simulink model "simTopLevel"  (R2016b)
settings: Solver=ode15s  StartTime=0.0  StopTime=2  RelTol=1e-3  EnableMultiTasking=on
InitFcn:
  | % minitaurParameters
model workspace (MAT data in the model file):
  IC = Simulink.Parameter
  IC.Value.Minitaur.IAq = -0.785398163397
  IC.Value.Minitaur.IAqDot = 0
  IC.Value.Minitaur.IBq = 0.785398163397
  IC.Value.Minitaur.IBqDot = 0
  IC.Value.Minitaur.IIAq = -0.785398163397
  IC.Value.Minitaur.IIAqDot = 0
  IC.Value.Minitaur.IIBq = 0.785398163397
  IC.Value.Minitaur.IIBqDot = 0
  IC.Value.Minitaur.IIIAq = -0.785398163397
  IC.Value.Minitaur.IIIAqDot = 0
  IC.Value.Minitaur.IIIBq = 0.785398163397
  IC.Value.Minitaur.IIIBqDot = 0
  IC.Value.Minitaur.IVAq = -0.785398163397
  IC.Value.Minitaur.IVAqDot = 0
  IC.Value.Minitaur.IVBq = 0.785398163397
  IC.Value.Minitaur.IVBqDot = 0
  IC.Value.Minitaur.ToeJointR = 1.57079632679
  IC.Value.Minitaur.ToeJointL = -1.57079632679
  IC.Value.Minitaur.Body.x = 0
  IC.Value.Minitaur.Body.y = -48
  IC.Value.Minitaur.Body.z = 0.7
  IC.Value.Minitaur.Body.xDot = 0
  IC.Value.Minitaur.Body.yDot = 0
  IC.Value.Minitaur.Body.zDot = 0
  IC.Value.Minitaur.Body.RotXZX = [0 3.14159265359 1.57079632679]
  IC.Value.Minitaur.Body.w = [0 0 0]
  IC.DataType = 'struct'
  IC.Dimensions = [1 1]
  controlParams = Simulink.Parameter
  controlParams.Value.jointPID.P = 6
  controlParams.Value.jointPID.I = 0.1
  controlParams.Value.jointPID.D = 0.07
  controlParams.Value.jointPID.N = 1000
  controlParams.Value.CPG.ForeRearLag = 1.57079632679
  controlParams.Value.CPG.Period = 1
  controlParams.Value.CPG.LRSyncFlag = 0
  controlParams.Value.FootImpedanceControl.r0 = -0.2
  controlParams.Value.FootImpedanceControl.rx = 0.04
  controlParams.Value.FootImpedanceControl.ry = 0.04
  controlParams.Value.FootImpedanceControl.thetaTilt = 0
  controlParams.DataType = 'struct'
  controlParams.Dimensions = [1 1]
  envParams = Simulink.Parameter
  envParams.Value.Ground.Width = 10
  envParams.Value.Ground.Length = 100
  envParams.Value.Ground.FrameDepth = 0.5
  envParams.Value.Contact.FootContactRadius = 0.0075
  envParams.Value.Contact.Stiffness = 10000
  envParams.Value.Contact.Damping = 1000
  envParams.Value.Contact.MuK = 0.75
  envParams.Value.Contact.MuS = 1
  envParams.Value.Contact.VelThresh = 0.01
  envParams.DataType = 'struct'
  envParams.Dimensions = [1 1]
  minitaurParams : Simulink.Parameter (value not decoded)
values from neighbouring files (symbols this model uses):
  controlParams = Simulink.Parameter(controlParams)    [minitaurParameters.m]
  envParams = Simulink.Parameter(envParams)    [minitaurParameters.m]
  IC = Simulink.Parameter(IC)    [minitaurParameters.m]
  minitaurParams = Simulink.Parameter(minitaurParams)    [minitaurParameters.m]
undefined symbols (not defined in the file or in its folder): Axis, Fn, ForeRearLag, Period, tau0, tau1, X, Y, Z
libraries: sm_lib x464, fl_lib x132, nesl_utility x41, Contact_Forces_Lib x28, simulink x13, simulink_extras x1
(part 1 of 13)
settings Model: SimulationMode=rapid-accelerator  Creator=Alexander  LastModifiedBy=Alexander
settings SolverCC: InitialStep=1e-12  MaxOrder=2  ZeroCrossAlgorithm=Adaptive  AlgebraicLoopSolver=LineSearch
settings DataIOCC: SaveFormat=StructureWithTime  SaveOutput=off  DSMLogging=off  SaveTime=off  SignalLoggingName=loggedSignals  ReturnWorkspaceOutputsName=simOut
settings OptimizationCC: DefaultParameterBehavior=Inlined  UseFloatMulNetSlope=on  InlineInvariantSignals=on  EfficientFloat2IntCast=on  EfficientMapNaN2IntZero=off  SimCompilerOptimization=on  AccelVerboseBuild=on
settings DebuggingCC: ReadBeforeWriteMsg=DisableAll  WriteAfterWriteMsg=DisableAll  WriteAfterReadMsg=DisableAll  MultiTaskDSMMsg=none  StrictBusMsg=ErrorOnBusTreatedAsVector  SFUnexpectedBacktrackingDiag=warning  SFNoUnconditionalDefaultTransitionDiag=warning  SFExecutionAtInitializationDiag=none
settings HardwareCC: TargetBitPerPointer=64  TargetBitPerSizeT=64  TargetBitPerPtrDiffT=64  TargetLongLongMode=on  TargetIntDivRoundTo=Zero  TargetEndianess=LittleEndian  TargetWordSize=64  TargetHWDeviceType=MATLAB Host
settings ModelReferenceCC: UpdateModelReferenceTargets=IfOutOfDate  ModelReferenceMinAlgLoopOccurrences=on
settings SFSimCC: SFSimEcho=off  SimBuildMode=sf_nonincremental_build
settings RTWCC: SystemTargetFile=rsim.tlc  TemplateMakefile=rsim_default_tmf  Description=Rapid Simulation Target  BuildConfiguration=Faster Runs  RTWCompilerOptimization=on
settings CodeAppCC: GenerateComments=off  MaxIdLength=128  SimulinkBlockComments=off
settings RSimTargetCC: TargetLangStandard=C99 (ISO)  ERTMultiwordTypeDef=System defined  ERTMultiwordLength=256  GeneratePreprocessorConditionals=Use local settings  CombineOutputUpdateFcns=on  MatFileLogging=off  SupportNonFinite=off  GRTInterface=off
settings ConfigComp: CovMetricSettings=dw  CovHtmlReporting=on  CovSaveCumulativeToWorkspaceVar=on  CovSaveSingleToWorkspaceVar=on  CovExternalEMLEnable=off
settings SimscapeCC: SimscapeLogSimulationStatistics=on  SimscapeLogLimitData=off
settings DiagnosticsConfigSet: SimMechanicsConflictingReferenceFrames=none  SimMechanicsRigidlyBoundBlock=none
settings ExplorerConfigSet: SimMechanicsOpenEditorOnUpdate=off  InternalSimMechanicsExplorerSettings="<ExplorerConfiguration><canonicalview>default</canonicalview><AnimationSetting><BasePlaybackSpeed>1.0</BasePlaybackSpeed><PlaybackSpeedFactor>0.125</PlaybackSpeedFactor></AnimationSetting><TilePanel><TileInfo><Tiles Columns=\"1\" Count=\"1\" Rows=\"1\"><Column Left=\"2\" Weight=\"1\"/><Column Left=\"1756\"/><Row Top=\"2\" Weight=\"1\"/><Row Top=\"912\"/><Tile Height=\"1\" Width=\"1\" X=\"0\" Y=\"0\"/></Tiles></TileInfo><SceneInfo><SceneViewer><BGColor><R>1</R><G>1</G><B>1</B></BGColor><Camera><DoPerspective>off</DoPerspective><Position><X>-52.933294827113023</X><Y>-19.442216136587813</Y><Z>35.583757754903054</Z></Position><Center><X>-14.397719012965357</X><Y>-39.827842104588491</Y><Z>10.080859987122921</Z></Center><Up><X>0.49923040919556116</X><Y>-0.12831156182763981</Y><Z>0.85691606452194846</Z></Up><ViewLimDist>1</ViewLimDist><YLim>0.49041337827292897</YLim><XLim>0.9498017148571154</XLim></Camera></SceneViewer></SceneInfo></TilePanel><MechEditorPanel><Cameras><Camera><Id>Camera1</Id><Value><Name>POV Camera</Name><NativeCamera><PositionTrackingFeature>POV_Camera.R</PositionTrackingFeature><CenterTrackingFeature>POV_Camera.R</CenterTrackingFeature><UpVectorTrackingFeature>POV_Camera.R</UpVectorTrackingFeature><CenterTrackingOrigin>off</CenterTrackingOrigin><CenterTrackingDirection>-Z</CenterTrackingDirection><UpVectorTrackingDirection>-Y</UpVectorTrackingDirection></NativeCamera></Value></Camera><Camera><Id>Camera2</Id><Value><Name>Side View</Name><NativeCamera><PositionTrackingFeature>Side_View_Camera.R</PositionTrackingFeature><CenterTrackingFeature>Body_Tracker.F</CenterTrackingFeature><UpVectorTrackingFeature>World1.W</UpVectorTrackingFeature><CenterTrackingOrigin>on</CenterTrackingOrigin><UpVectorTrackingDirection>+Z</UpVectorTrackingDirection></NativeCamera></Value></Camera></Cameras><GfxPanelCameraMap/><VideoCreator><PlaybackSpeedRatio>1.0</PlaybackSpeedRatio><FrameRate>30</FrameRate><VideoFormat>Motion JPEG AVI</VideoFormat><FrameSize>auto</FrameSize></VideoCreator></MechEditorPanel></ExplorerConfiguration>"

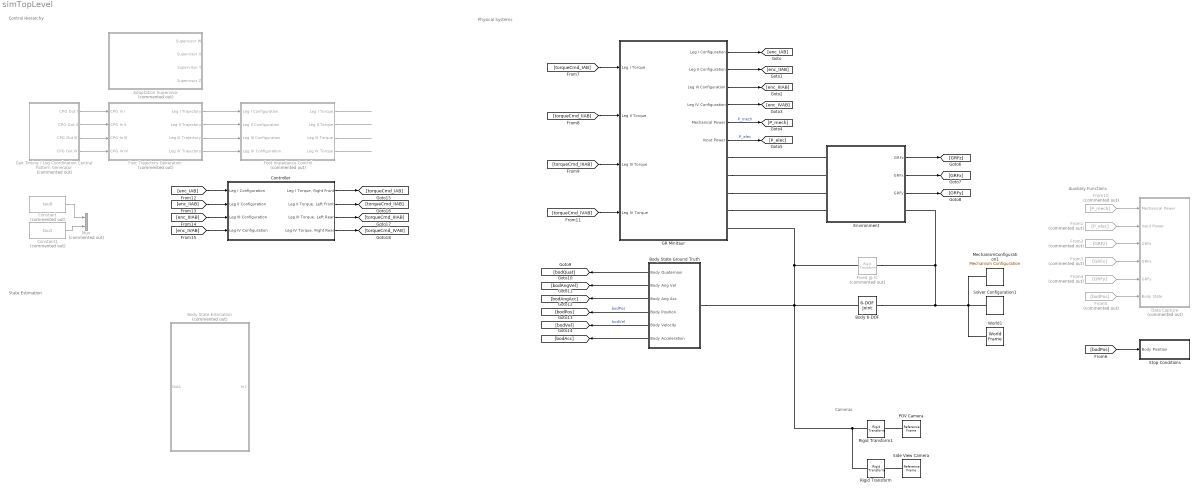
== system simTopLevel ==
  note: Physical Systems
  note: Control Hierarchy
  note: Auxiliary Functions
  note: Cameras
  note: State Estimation
  Adaptation Supervisor : Subsystem  Commented=on
  Body 6-DOF : sm_lib/Joints/6-DOF Joint  SenseConstraintForce=off  SenseConstraintForceX=off  SenseConstraintForceY=off  SenseConstraintForceZ=off  SenseConstraintTorque=off  SenseConstraintTorqueX=off  SenseConstraintTorqueY=off  SenseConstraintTorqueZ=off  SenseTotalForce=off  SenseTotalForceX=off  SenseTotalForceY=off  SenseTotalForceZ=off  SenseTotalTorque=off  SenseTotalTorqueX=off  SenseTotalTorqueY=off  SenseTotalTorqueZ=off  CompositeWrenchDir=FollowerOnBase  CompositeWrenchFrame=BaseFrame  PxEquilibriumPosition=0  PxEquilibriumPositionUnits=m  PxSpringStiffness=0  PxSpringStiffnessUnits=N/m  PxDampingCoefficient=0  PxDampingCoefficientUnits=N/(m/s)  PxTorqueActuationMode=NoTorque  PxMotionActuationMode=ComputedMotion  PxSensePosition=off  PxSenseVelocity=off  PxSenseAcceleration=off  PxSenseTorqueForce=off  PxPositionTargetSpecify=on  PxPositionTargetPriority=High  PxPositionTargetValue=IC.Minitaur.Body.x  PxPositionTargetValueUnits=m  PxVelocityTargetSpecify=on  PxVelocityTargetPriority=High  PxVelocityTargetValue=IC.Minitaur.Body.xDot  PxVelocityTargetValueUnits=m/s  PyEquilibriumPosition=0  PyEquilibriumPositionUnits=m  PySpringStiffness=0  PySpringStiffnessUnits=N/m  PyDampingCoefficient=0  PyDampingCoefficientUnits=N/(m/s)  PyTorqueActuationMode=NoTorque  PyMotionActuationMode=ComputedMotion  PySensePosition=off  PySenseVelocity=off  PySenseAcceleration=off  PySenseTorqueForce=off  PyPositionTargetSpecify=on  PyPositionTargetPriority=High  PyPositionTargetValue=IC.Minitaur.Body.y  PyPositionTargetValueUnits=m  PyVelocityTargetSpecify=on  PyVelocityTargetPriority=High  PyVelocityTargetValue=IC.Minitaur.Body.yDot  PyVelocityTargetValueUnits=m/s  PzEquilibriumPosition=1  PzEquilibriumPositionUnits=m  PzSpringStiffness=0  PzSpringStiffnessUnits=N/m  PzDampingCoefficient=0  PzDampingCoefficientUnits=N/(m/s)  PzTorqueActuationMode=NoTorque  PzMotionActuationMode=ComputedMotion  PzSensePosition=off  PzSenseVelocity=off  PzSenseAcceleration=off  PzSenseTorqueForce=off  PzPositionTargetSpecify=on  PzPositionTargetPriority=High  PzPositionTargetValue=IC.Minitaur.Body.z  PzPositionTargetValueUnits=m  PzVelocityTargetSpecify=on  PzVelocityTargetPriority=High  PzVelocityTargetValue=IC.Minitaur.Body.zDot  PzVelocityTargetValueUnits=m/s  SphDefPosRotationMethod=None  SphDefPosRotationAngleUnits=deg  SphDefPosRotationStandardAxis=+Z  SphDefPosRotationAngle=0.0  SphDefPosRotationArbitraryAxis=[0 0 1]  SphDefPosFollAlignAxisA=+X  SphDefPosBaseAlignAxisA=+Y  SphDefPosFollAlignAxisB=+Y  SphDefPosBaseAlignAxisB=+Z  SphDefPosRotationSequenceAxes=FollowerAxes  SphDefPosRotationSequence=XYX  SphDefPosRotationSequenceAngles=[0 0 0]  SphDefPosRotationSequenceAnglesUnits=deg  SphDefPosRotationMatrix=[1 0 0; 0 1 0; 0 0 1]  SphEqPosRotationMethod=None  SphEqPosRotationAngleUnits=deg  SphEqPosRotationStandardAxis=+Z  SphEqPosRotationAngle=0.0  SphEqPosRotationArbitraryAxis=[0 0 1]  SphEqPosFollAlignAxisA=+X  SphEqPosBaseAlignAxisA=+Y  SphEqPosFollAlignAxisB=+Y  SphEqPosBaseAlignAxisB=+Z  SphEqPosRotationSequenceAxes=FollowerAxes  SphEqPosRotationSequence=XYX  SphEqPosRotationSequenceAngles=[0 0 0]  SphEqPosRotationSequenceAnglesUnits=deg  SphEqPosRotationMatrix=[1 0 0; 0 1 0; 0 0 1]  SphSpringStiffness=0  SphSpringStiffnessUnits=N*m/deg  SphDampingCoefficient=0  SphDampingCoefficientUnits=N*m/(deg/s)  SphActuateTorqueX=off  SphActuateTorqueY=off  SphActuateTorqueZ=off  SphActuateTorque=off  SphTorqueActuationMode=NoTorque  SphMotionActuationMode=ComputedMotion  SphActuationFrame=BaseFrame  SphSensePosition=off  SphSenseVelocityX=off  SphSenseVelocityY=off  SphSenseVelocityZ=off  SphSenseVelocity=off  SphSenseAccelerationX=off  SphSenseAccelerationY=off  SphSenseAccelerationZ=off  SphSenseAcceleration=off  SphSenseTorqueX=off  SphSenseTorqueY=off  SphSenseTorqueZ=off  SphSenseTorqueForce=off  SphSensingFrame=BaseFrame  SphPositionTargetRotationMethod=RotationSequence  SphPositionTargetRotationAngleUnits=deg  SphPositionTargetRotationStandardAxis=+Z  SphPositionTargetRotationAngle=0.0  SphPositionTargetRotationArbitraryAxis=[0 0 1]  SphPositionTargetFollAlignAxisA=+X  SphPositionTargetBaseAlignAxisA=+Y  SphPositionTargetFollAlignAxisB=+Y  SphPositionTargetBaseAlignAxisB=+Z  SphPositionTargetRotationSequenceAxes=BaseAxes  SphPositionTargetRotationSequence=XZX  SphPositionTargetRotationSequenceAngles=IC.Minitaur.Body.RotXZX  SphPositionTargetRotationSequenceAnglesUnits=rad  SphPositionTargetRotationMatrix=[1 0 0; 0 1 0; 0 0 1]  SphPositionTargetSpecify=on  SphPositionTargetPriority=High  SphVelocityTargetValue=IC.Minitaur.Body.w  SphVelocityTargetValueUnits=rad/s  SphVelocityTargetSpecify=on  SphVelocityTargetPriority=High  SphVelocityTargetInFollowerFrame=off
  Body State Estimation : Subsystem  Commented=on
  Body State Ground Truth : Subsystem
  Constant : Constant  Commented=on  Value=tau0
  Constant1 : Constant  Commented=on  Value=tau1
  Controller : Subsystem
  Data Capture : Subsystem  Commented=on
  Environment : Subsystem
  Fixed @ IC : sm_lib/Frames and Transforms/Rigid Transform  Commented=on  TranslationMethod=Cartesian  TranslationStandardOffset=0  TranslationLengthUnit=m  TranslationStandardAxis=+Z  TranslationCartesianOffset=[IC.Minitaur.Body.x IC.Minitaur.Body.y IC.Minitaur.Body.z + 0.5]  TranslationROffset=0  TranslationROffsetUnits=m  TranslationZOffset=0  TranslationZOffsetUnits=m  TranslationThetaOffset=0  TranslationThetaOffsetUnits=deg  RotationMethod=RotationSequence  RotationAngleUnits=deg  RotationStandardAxis=+Z  RotationAngle=0.0  RotationArbitraryAxis=[0 0 1]  FollAlignAxisA=+X  BaseAlignAxisA=+Y  FollAlignAxisB=+Y  BaseAlignAxisB=+Z  RotationSequenceAxes=BaseAxes  RotationSequence=XZX  RotationSequenceAngles=IC.Minitaur.Body.RotXZX  RotationSequenceAnglesUnits=rad  RotationMatrix=[1 0 0; 0 1 0; 0 0 1]
  Foot Impedance Control : Subsystem  Commented=on
  Foot Trajectory Generation : Subsystem  Commented=on
  From1 : From  Commented=on  GotoTag=P_elec
  From10 : From  Commented=on  GotoTag=P_mech
  From2 : From  Commented=on  GotoTag=GRFz
  From3 : From  Commented=on  GotoTag=GRFx
  From4 : From  Commented=on  GotoTag=GRFy
  From5 : From  Commented=on  GotoTag=bodPos
  GR Minitaur : Subsystem
  Gait Timing / Leg Coordination Central Pattern Generator : Subsystem  Commented=on
  MechanismConfiguration1 : sm_lib/Utilities/Mechanism Configuration  UniformGravity=Constant  GravityVector="[0  0 -9.81]"  GravityUnits=m/s^2  LinearizationDelta=0.001
  Mux : Mux  Commented=on  Inputs=2
  POV Camera : sm_lib/Frames and Transforms/Reference Frame
  Rigid Transform : sm_lib/Frames and Transforms/Rigid Transform  TranslationMethod=Cartesian  TranslationStandardOffset=envParams.Ground.FrameDepth/2  TranslationLengthUnit=m  TranslationStandardAxis=+X  TranslationCartesianOffset=[-1 0 0]  TranslationROffset=0  TranslationROffsetUnits=m  TranslationZOffset=0  TranslationZOffsetUnits=m  TranslationThetaOffset=0  TranslationThetaOffsetUnits=deg  RotationMethod=None  RotationAngleUnits=deg  RotationStandardAxis=+Z  RotationAngle=0.0  RotationArbitraryAxis=[0 0 1]  FollAlignAxisA=+X  BaseAlignAxisA=+Y  FollAlignAxisB=+Y  BaseAlignAxisB=+Z  RotationSequenceAxes=FollowerAxes  RotationSequence=XYX  RotationSequenceAngles=[0 0 0]  RotationSequenceAnglesUnits=deg  RotationMatrix=[1 0 0; 0 1 0; 0 0 1]
  Rigid Transform1 : sm_lib/Frames and Transforms/Rigid Transform  TranslationMethod=Cartesian  TranslationStandardOffset=0  TranslationLengthUnit=m  TranslationStandardAxis=+Z  TranslationCartesianOffset=[0 -0.1 -0.125]  TranslationROffset=0  TranslationROffsetUnits=m  TranslationZOffset=0  TranslationZOffsetUnits=m  TranslationThetaOffset=0  TranslationThetaOffsetUnits=deg  RotationMethod=None  RotationAngleUnits=deg  RotationStandardAxis=+Z  RotationAngle=0.0  RotationArbitraryAxis=[0 0 1]  FollAlignAxisA=+X  BaseAlignAxisA=+Y  FollAlignAxisB=+Y  BaseAlignAxisB=+Z  RotationSequenceAxes=FollowerAxes  RotationSequence=XYX  RotationSequenceAngles=[0 0 0]  RotationSequenceAnglesUnits=deg  RotationMatrix=[1 0 0; 0 1 0; 0 0 1]
  Side View Camera : sm_lib/Frames and Transforms/Reference Frame
  Solver Configuration1 : nesl_utility/Solver Configuration  PhysicalDomain=network_engine_domain  SubClassName=solver  LeftPortType=input  RightPortType=generic  Accelerate=off  Tones=[]  Harmonics=[]  SimulateNoise=off  Profile=off  UseLocalSampling=off  EnableSwitchedLinearOptims=on  FrequencyDomain=off  UseCCode=off  RelTol=0.001  AbsTol=1e-06  MinStep=1e-09  ToWorkspace=off  RevertToSquareIcSolve=off  NumHomotopyIterations=100  PhasorMode=off  PhasorModeNumHarmonics=1  OverrideAbsTol=off  DoDC=off  ResidualTolerance=1e-09  UseLocalSolver=off  LocalSolverChoice=NE_BACKWARD_EULER_ADVANCER  LocalSolverSampleTime=0.001  DoFixedCost=off  MaxNonlinIter=3  MaxModeIter=2  LinearAlgebra=Sparse  DelaysMemoryBudget=1024  AutomaticFiltering=on  FilteringTimeConstant=0.001
  Stop Conditions : Subsystem
  World1 : sm_lib/Frames and Transforms/World Frame
  wires:
  GR Minitaur/1(Leg I Configuration) -> [enc_IAB]
  GR Minitaur/2(Leg II Configuration) -> [enc_IIAB]
  GR Minitaur/3(Leg III Configuration) -> [enc_IIIAB]
  GR Minitaur/4(Leg IV Configuration) -> [enc_IVAB]
  GR Minitaur/5(Mechanical Power) -> [P_mech]  "P_mech"
  GR Minitaur/6(Input Power) -> [P_elec]  "P_elec"
  From10/1 -> Data Capture/1(Mechanical Power)
  From1/1 -> Data Capture/2(Input Power)
  From2/1 -> Data Capture/3(GRFz)
  From3/1 -> Data Capture/4(GRFx)
  From4/1 -> Data Capture/5(GRFy)
  From5/1 -> Data Capture/6(Body State)
  Environment/1(GRFz) -> [GRFz]
  Environment/2(GRFx) -> [GRFx]
  Environment/3(GRFy) -> [GRFy]
  [bodPos] -> Stop Conditions/1(Body Position)
  [torqueCmd_IAB] -> GR Minitaur/1(Leg I Torque)
  [torqueCmd_IIAB] -> GR Minitaur/2(Leg II Torque)
  [torqueCmd_IIIAB] -> GR Minitaur/3(Leg III Torque)
  [torqueCmd_IVAB] -> GR Minitaur/4(Leg IV Torque)
  Body State Ground Truth/1(Body Quaternion) -> [bodQuat]
  Body State Ground Truth/2(Body Ang Vel) -> [bodAngVel]
  Body State Ground Truth/3(Body Ang Acc) -> [bodAngAcc]
  Body State Ground Truth/5(Body Velocity) -> [bodVel]  "bodVel"
  Body State Ground Truth/6(Body Acceleration) -> [bodAcc]
  Body State Ground Truth/4(Body Position) -> [bodPos]  "bodPos"
  Gait Timing / Leg Coordination Central Pattern Generator/1(CPG Out I) -> Foot Trajectory Generation/1(CPG In I)
  Gait Timing / Leg Coordination Central Pattern Generator/2(CPG Out II) -> Foot Trajectory Generation/2(CPG In II)
  Gait Timing / Leg Coordination Central Pattern Generator/3(CPG Out III) -> Foot Trajectory Generation/3(CPG In III)
  Gait Timing / Leg Coordination Central Pattern Generator/4(CPG Out IV) -> Foot Trajectory Generation/4(CPG In IV)
  Foot Trajectory Generation/1(Leg I Trajectory) -> Foot Impedance Control/1(Leg I Configuration)
  Foot Trajectory Generation/2(Leg II Trajectory) -> Foot Impedance Control/2(Leg II Configuration)
  Foot Trajectory Generation/3(Leg III Trajectory) -> Foot Impedance Control/3(Leg III Configuration)
  Foot Trajectory Generation/4(Leg IV Trajectory) -> Foot Impedance Control/4(Leg IV Configuration)
  Foot Impedance Control/1(Leg I Torque) -> ?
  Foot Impedance Control/2(Leg II Torque) -> ?
  Foot Impedance Control/4(Leg IV Torque) -> ?
  Foot Impedance Control/3(Leg III Torque) -> ?
  Constant1/1 -> Mux/2
  Constant/1 -> Mux/1
  Controller/1("Leg I Torque, Right Front") -> [torqueCmd_IAB]
  Controller/2("Leg II Torque, Left Front") -> [torqueCmd_IIAB]
  Controller/4("Leg IV Torque, Right Rear") -> [torqueCmd_IVAB]
  Controller/3("Leg III Torque, Left Rear") -> [torqueCmd_IIIAB]
  [enc_IAB] -> Controller/1(Leg I Configuration)
  [enc_IIAB] -> Controller/2(Leg II Configuration)
  [enc_IIIAB] -> Controller/3(Leg III Configuration)
  [enc_IVAB] -> Controller/4(Leg IV Configuration)
  connections:
  MechanismConfiguration1/RConn1 -- Solver Configuration1/RConn1 -- World1/RConn1 -- Fixed @ IC/LConn1 -- Environment/RConn1 -- Body 6-DOF/LConn1
  GR Minitaur/RConn4 -- Environment/LConn4
  GR Minitaur/RConn3 -- Environment/LConn3
  GR Minitaur/RConn2 -- Environment/LConn2
  GR Minitaur/RConn1 -- Environment/LConn1
  Rigid Transform/LConn1 -- Body State Ground Truth/LConn1 -- GR Minitaur/RConn5 -- Fixed @ IC/RConn1 -- Body 6-DOF/RConn1 -- Rigid Transform1/LConn1
  Side View Camera/RConn1 -- Rigid Transform/RConn1
  POV Camera/RConn1 -- Rigid Transform1/RConn1

== system simTopLevel/Adaptation Supervisor ==
  Constant{,1..3} (4 alike) : Constant
  Supervisor W : Outport
  Supervisor X : Outport  Port=2
  Supervisor Y : Outport  Port=3
  Supervisor Z : Outport  Port=4
  wires:
  Constant/1 -> Supervisor W/1
  Constant3/1 -> Supervisor Z/1
  Constant2/1 -> Supervisor Y/1
  Constant1/1 -> Supervisor X/1

== system simTopLevel/Body State Estimation ==
  In1 : Inport
  Out1 : Outport
  wires:
  In1/1 -> Out1/1

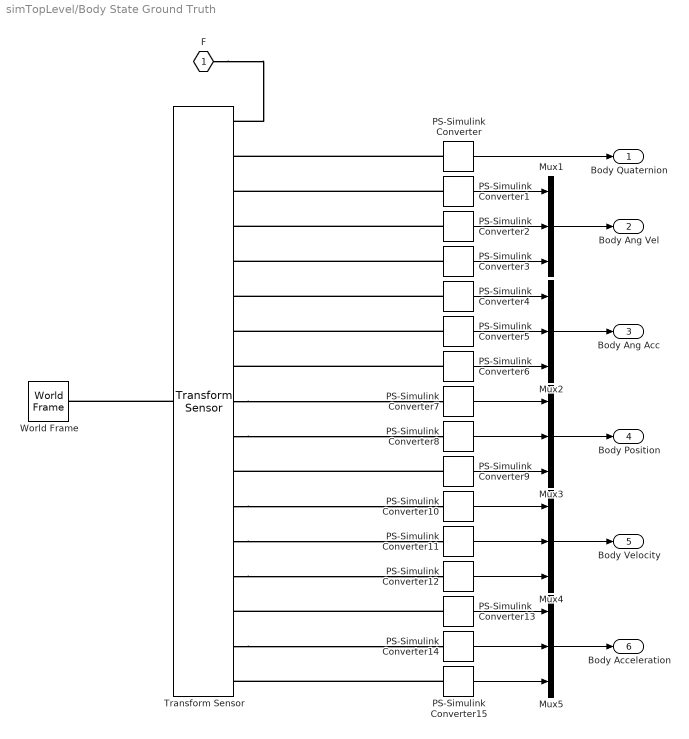
== system simTopLevel/Body State Ground Truth ==
  Mux{1..5} (5 alike) : Mux  Inputs=3
  PS-Simulink Converter : nesl_utility/PS-Simulink Converter  PhysicalDomain=network_engine_domain  SubClassName=ps_output  LeftPortType=input  RightPortType=output  PseudoPeriodic=off  Frequencies=[]  Unit=1  AffineConversion=off
  PS-Simulink Converter1 : nesl_utility/PS-Simulink Converter  PhysicalDomain=network_engine_domain  SubClassName=ps_output  LeftPortType=input  RightPortType=output  PseudoPeriodic=off  Frequencies=[]  Unit=rad/s  AffineConversion=off
  PS-Simulink Converter10 : nesl_utility/PS-Simulink Converter  PhysicalDomain=network_engine_domain  SubClassName=ps_output  LeftPortType=input  RightPortType=output  PseudoPeriodic=off  Frequencies=[]  Unit=m/s  AffineConversion=off
  PS-Simulink Converter11 : nesl_utility/PS-Simulink Converter  PhysicalDomain=network_engine_domain  SubClassName=ps_output  LeftPortType=input  RightPortType=output  PseudoPeriodic=off  Frequencies=[]  Unit=m/s  AffineConversion=off
  PS-Simulink Converter12 : nesl_utility/PS-Simulink Converter  PhysicalDomain=network_engine_domain  SubClassName=ps_output  LeftPortType=input  RightPortType=output  PseudoPeriodic=off  Frequencies=[]  Unit=m/s  AffineConversion=off
  PS-Simulink Converter13 : nesl_utility/PS-Simulink Converter  PhysicalDomain=network_engine_domain  SubClassName=ps_output  LeftPortType=input  RightPortType=output  PseudoPeriodic=off  Frequencies=[]  Unit=m/s^2  AffineConversion=off
  PS-Simulink Converter14 : nesl_utility/PS-Simulink Converter  PhysicalDomain=network_engine_domain  SubClassName=ps_output  LeftPortType=input  RightPortType=output  PseudoPeriodic=off  Frequencies=[]  Unit=m/s^2  AffineConversion=off
  PS-Simulink Converter15 : nesl_utility/PS-Simulink Converter  PhysicalDomain=network_engine_domain  SubClassName=ps_output  LeftPortType=input  RightPortType=output  PseudoPeriodic=off  Frequencies=[]  Unit=m/s^2  AffineConversion=off
  PS-Simulink Converter2 : nesl_utility/PS-Simulink Converter  PhysicalDomain=network_engine_domain  SubClassName=ps_output  LeftPortType=input  RightPortType=output  PseudoPeriodic=off  Frequencies=[]  Unit=rad/s  AffineConversion=off
  PS-Simulink Converter3 : nesl_utility/PS-Simulink Converter  PhysicalDomain=network_engine_domain  SubClassName=ps_output  LeftPortType=input  RightPortType=output  PseudoPeriodic=off  Frequencies=[]  Unit=rad/s  AffineConversion=off
  PS-Simulink Converter4 : nesl_utility/PS-Simulink Converter  PhysicalDomain=network_engine_domain  SubClassName=ps_output  LeftPortType=input  RightPortType=output  PseudoPeriodic=off  Frequencies=[]  Unit=rad/s^2  AffineConversion=off
  PS-Simulink Converter5 : nesl_utility/PS-Simulink Converter  PhysicalDomain=network_engine_domain  SubClassName=ps_output  LeftPortType=input  RightPortType=output  PseudoPeriodic=off  Frequencies=[]  Unit=rad/s^2  AffineConversion=off
  PS-Simulink Converter6 : nesl_utility/PS-Simulink Converter  PhysicalDomain=network_engine_domain  SubClassName=ps_output  LeftPortType=input  RightPortType=output  PseudoPeriodic=off  Frequencies=[]  Unit=rad/s^2  AffineConversion=off
  PS-Simulink Converter7 : nesl_utility/PS-Simulink Converter  PhysicalDomain=network_engine_domain  SubClassName=ps_output  LeftPortType=input  RightPortType=output  PseudoPeriodic=off  Frequencies=[]  Unit=m  AffineConversion=off
  PS-Simulink Converter8 : nesl_utility/PS-Simulink Converter  PhysicalDomain=network_engine_domain  SubClassName=ps_output  LeftPortType=input  RightPortType=output  PseudoPeriodic=off  Frequencies=[]  Unit=m  AffineConversion=off
  PS-Simulink Converter9 : nesl_utility/PS-Simulink Converter  PhysicalDomain=network_engine_domain  SubClassName=ps_output  LeftPortType=input  RightPortType=output  PseudoPeriodic=off  Frequencies=[]  Unit=m  AffineConversion=off
  Transform Sensor : sm_lib/Frames and Transforms/Transform Sensor  MeasurementFrame=World  SenseAngle=off  SenseAxis=off  SenseAngle1=off  SenseAngle2=off  SenseAngle3=off  SenseQ=on  SenseR=off  SenseOmegaX=on  SenseOmegaY=on  SenseOmegaZ=on  SenseOmega1=off  SenseOmega2=off  SenseOmega3=off  SenseQDot=off  SenseRDot=off  SenseAlphaX=on  SenseAlphaY=on  SenseAlphaZ=on  SenseAlpha1=off  SenseAlpha2=off  SenseAlpha3=off  SenseQDDot=off  SenseRDDot=off  SenseX=on  SenseY=on  SenseZ=on  SenseRad=off  SenseAzim=off  SenseDist=off  SenseInc=off  SenseXDot=on  SenseYDot=on  SenseZDot=on  SenseRadDot=off  SenseAzimDot=off  SenseDistDot=off  SenseIncDot=off  SenseXDDot=on  SenseYDDot=on  SenseZDDot=on  SenseRadDDot=off  SenseAzimDDot=off  SenseDistDDot=off  SenseIncDDot=off
  World Frame : sm_lib/Frames and Transforms/World Frame
  F : PMIOPort  Port=1  Side=Left
  Body Quaternion : Outport
  Body Ang Vel : Outport  Port=2
  Body Ang Acc : Outport  Port=3
  Body Position : Outport  Port=4
  Body Velocity : Outport  Port=5
  Body Acceleration : Outport  Port=6
  wires:
  PS-Simulink Converter3/1 -> Mux1/3
  PS-Simulink Converter2/1 -> Mux1/2
  PS-Simulink Converter1/1 -> Mux1/1
  PS-Simulink Converter/1 -> Body Quaternion/1
  Mux1/1 -> Body Ang Vel/1
  PS-Simulink Converter4/1 -> Mux2/1
  PS-Simulink Converter5/1 -> Mux2/2
  Mux2/1 -> Body Ang Acc/1
  PS-Simulink Converter6/1 -> Mux2/3
  PS-Simulink Converter7/1 -> Mux3/1
  PS-Simulink Converter8/1 -> Mux3/2
  PS-Simulink Converter9/1 -> Mux3/3
  Mux3/1 -> Body Position/1
  PS-Simulink Converter10/1 -> Mux4/1
  PS-Simulink Converter11/1 -> Mux4/2
  PS-Simulink Converter12/1 -> Mux4/3
  Mux4/1 -> Body Velocity/1
  PS-Simulink Converter13/1 -> Mux5/1
  PS-Simulink Converter14/1 -> Mux5/2
  PS-Simulink Converter15/1 -> Mux5/3
  Mux5/1 -> Body Acceleration/1
  connections:
  PS-Simulink Converter1/LConn1 -- Transform Sensor/RConn3
  PS-Simulink Converter5/LConn1 -- Transform Sensor/RConn7
  PS-Simulink Converter4/LConn1 -- Transform Sensor/RConn6
  F/RConn1 -- Transform Sensor/RConn1
  PS-Simulink Converter/LConn1 -- Transform Sensor/RConn2
  Transform Sensor/LConn1 -- World Frame/RConn1
  PS-Simulink Converter2/LConn1 -- Transform Sensor/RConn4
  PS-Simulink Converter3/LConn1 -- Transform Sensor/RConn5
  PS-Simulink Converter6/LConn1 -- Transform Sensor/RConn8
  Transform Sensor/RConn9 -- PS-Simulink Converter7/LConn1
  PS-Simulink Converter9/LConn1 -- Transform Sensor/RConn11
  Transform Sensor/RConn10 -- PS-Simulink Converter8/LConn1
  Transform Sensor/RConn12 -- PS-Simulink Converter10/LConn1
  Transform Sensor/RConn13 -- PS-Simulink Converter11/LConn1
  Transform Sensor/RConn14 -- PS-Simulink Converter12/LConn1
  PS-Simulink Converter13/LConn1 -- Transform Sensor/RConn15
  PS-Simulink Converter15/LConn1 -- Transform Sensor/RConn17
  Transform Sensor/RConn16 -- PS-Simulink Converter14/LConn1

== system simTopLevel/Controller ==
  Leg I Configuration : Inport  PortDimensions=2
  Leg II Configuration : Inport  Port=2  PortDimensions=2
  Leg III Configuration : Inport  Port=3  PortDimensions=2
  Leg IV Configuration : Inport  Port=4  PortDimensions=2
  Subsystem1 : Subsystem
  Subsystem2 : Subsystem
  Subsystem3 : Subsystem
  Subsystem4 : Subsystem
  Trajectory Planner : Subsystem
  "Leg I Torque, Right Front" : Outport
  "Leg II Torque, Left Front" : Outport  Port=2
  "Leg III Torque, Left Rear" : Outport  Port=3
  "Leg IV Torque, Right Rear" : Outport  Port=4
  wires:
  Trajectory Planner/1(Foot I Trajectory [psi L]) -> Subsystem4/1(Path Trajectory)
  Leg I Configuration/1 -> Subsystem4/2(Current leg state)  "[theta_AI theta_BI] Nm"
  Subsystem4/1(Leg Torque) -> "Leg I Torque, Right Front"/1
  Trajectory Planner/2(Foot II Trajectory [psi L]) -> Subsystem1/1(Path Trajectory)
  Trajectory Planner/3(Foot III Trajectory [psi L]) -> Subsystem2/1(Path Trajectory)
  Trajectory Planner/4(Foot IV Trajectory [psi L]) -> Subsystem3/1(Path Trajectory)
  Leg II Configuration/1 -> Subsystem1/2(Current leg state)  "[Tau_IIA Tau_IIB] Nm"
  Leg III Configuration/1 -> Subsystem2/2(Current leg state)  "[Tau_IIIA Tau_IIIB] Nm"
  Leg IV Configuration/1 -> Subsystem3/2(Current leg state)  "[Tau_IVA Tau_IVB] Nm"
  Subsystem1/1(Leg Torque) -> "Leg II Torque, Left Front"/1
  Subsystem2/1(Leg Torque) -> "Leg III Torque, Left Rear"/1
  Subsystem3/1(Leg Torque) -> "Leg IV Torque, Right Rear"/1

== system simTopLevel/Data Capture ==
  Mechanical Power : Inport
  Input Power : Inport  Port=2
  GRFz : Inport  Port=3
  GRFx : Inport  Port=4
  GRFy : Inport  Port=5
  Body State : Inport  Port=6
  To Workspace : ToWorkspace  VariableName=P_mech  SaveFormat=Structure With Time  SampleTime=-1
  To Workspace1 : ToWorkspace  VariableName=body_state  SaveFormat=Structure With Time  SampleTime=-1
  To Workspace2 : ToWorkspace  VariableName=P_in  SaveFormat=Structure With Time  SampleTime=-1
  To Workspace3 : ToWorkspace  VariableName=GRF_z  SaveFormat=Structure With Time  SampleTime=-1
  To Workspace4 : ToWorkspace  VariableName=GRF_y  SaveFormat=Structure With Time  SampleTime=-1
  To Workspace5 : ToWorkspace  VariableName=GRF_x  SaveFormat=Structure With Time  SampleTime=-1
  wires:
  Body State/1 -> To Workspace1/1  "body_state"
  Mechanical Power/1 -> To Workspace/1  "P_mech"
  Input Power/1 -> To Workspace2/1  "P_in"
  GRFz/1 -> To Workspace3/1  "GRFz"
  GRFy/1 -> To Workspace4/1  "GRFy"
  GRFx/1 -> To Workspace5/1  "GRFx"

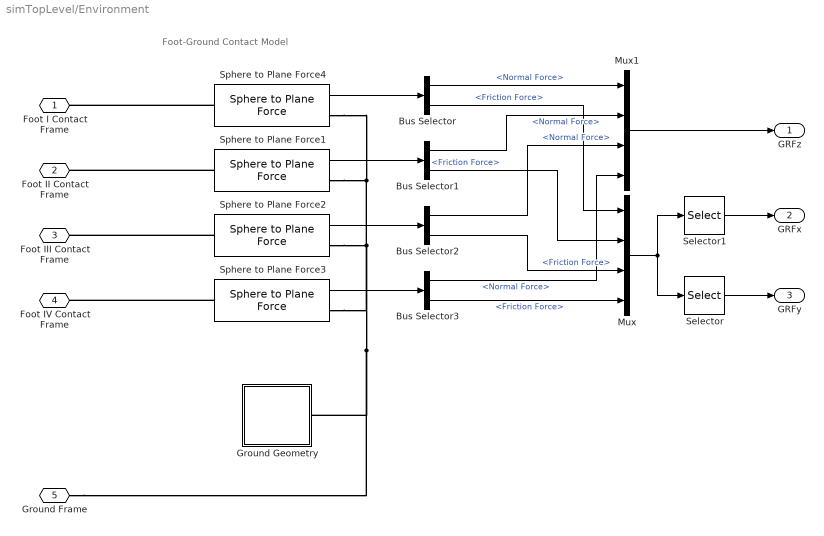
== system simTopLevel/Environment ==
  note: Foot-Ground Contact Model
  Bus Selector{,1..3} (4 alike) : BusSelector  OutputSignals=Normal Force,Friction Force
  Ground Geometry : Subsystem  mask(Ground (Track) Model){}
      mask help: Models the ground as a rigid body with a given reference frame.
  Mux : Mux
  Mux1 : Mux
  Selector : Selector  IndexMode=Zero-based  InputPortWidth=12  IndexOptions=Index vector (dialog)  Indices=[1:3:12]  OutputSizes=1
  Selector1 : Selector  IndexMode=Zero-based  InputPortWidth=12  IndexOptions=Index vector (dialog)  Indices=[2:3:12]  OutputSizes=1
  Sphere to Plane Force{1..4} (4 alike) : Contact_Forces_Lib/3D/Sphere to Plane Force  sphere_rad=envParams.Contact.FootContactRadius  plane_lenx=envParams.Ground.Width  plane_leny=envParams.Ground.Length  plane_depth=envParams.Ground.FrameDepth  force_law=Linear  k_contact=envParams.Contact.Stiffness  b_contact=envParams.Contact.Damping  pen_full_damp_F=1e-4  pen_exponent=1  custom_param_1=1  custom_param_2=1  friction_law=Stick-Slip Continuous  mu_kinetic=envParams.Contact.MuK  mu_static=envParams.Contact.MuS  v_thr=envParams.Contact.VelThresh
  Foot I Contact Frame : PMIOPort  Port=1  Side=Left
  Foot II Contact Frame : PMIOPort  Port=2  Side=Left
  Foot III Contact Frame : PMIOPort  Port=3  Side=Left
  Foot IV Contact Frame : PMIOPort  Port=4  Side=Left
  Ground Frame : PMIOPort  Port=5  Side=Right
  GRFz : Outport
  GRFx : Outport  Port=2
  GRFy : Outport  Port=3
  wires:
  Sphere to Plane Force3/1 -> Bus Selector3/1
  Sphere to Plane Force4/1 -> Bus Selector/1
  Sphere to Plane Force1/1 -> Bus Selector1/1
  Sphere to Plane Force2/1 -> Bus Selector2/1
  Bus Selector/1 -> Mux1/1  "<Normal Force>"
  Bus Selector/2 -> Mux/1  "<Friction Force>"
  Bus Selector1/1 -> Mux1/2  "<Normal Force>"
  Bus Selector1/2 -> Mux/2  "<Friction Force>"
  Bus Selector2/1 -> Mux1/3  "<Normal Force>"
  Bus Selector2/2 -> Mux/3  "<Friction Force>"
  Bus Selector3/1 -> Mux1/4  "<Normal Force>"
  Bus Selector3/2 -> Mux/4  "<Friction Force>"
  Mux1/1 -> GRFz/1
  Mux/1 -> Selector1/1, Selector/1
  Selector/1 -> GRFy/1
  Selector1/1 -> GRFx/1
  connections:
  Sphere to Plane Force1/RConn1 -- Sphere to Plane Force4/RConn1 -- Sphere to Plane Force2/RConn1 -- Sphere to Plane Force3/RConn1 -- Ground Frame/RConn1 -- Ground Geometry/RConn1
  Sphere to Plane Force4/LConn1 -- Foot I Contact Frame/RConn1
  Sphere to Plane Force3/LConn1 -- Foot IV Contact Frame/RConn1
  Sphere to Plane Force2/LConn1 -- Foot III Contact Frame/RConn1
  Sphere to Plane Force1/LConn1 -- Foot II Contact Frame/RConn1

== system simTopLevel/Foot Impedance Control ==
  Leg I Configuration : Inport  PortDimensions=2
  Leg II Configuration : Inport  Port=2  PortDimensions=2
  Leg III Configuration : Inport  Port=3  PortDimensions=2
  Leg IV Configuration : Inport  Port=4  PortDimensions=2
  Constant{,1..3} (4 alike) : Constant  Value=[0 0]
  Terminator{,1..3} (4 alike) : Terminator
  Leg I Torque : Outport
  Leg II Torque : Outport  Port=2
  Leg III Torque : Outport  Port=3
  Leg IV Torque : Outport  Port=4
  wires:
  Leg I Configuration/1 -> Terminator/1  "[rad rad]"
  Constant/1 -> Leg I Torque/1  "[Nm Nm]"
  Leg II Configuration/1 -> Terminator1/1  "[rad rad]"
  Leg III Configuration/1 -> Terminator2/1  "[rad rad]"
  Leg IV Configuration/1 -> Terminator3/1  "[rad rad]"
  Constant1/1 -> Leg II Torque/1  "[Nm Nm]"
  Constant2/1 -> Leg III Torque/1  "[Nm Nm]"
  Constant3/1 -> Leg IV Torque/1  "[Nm Nm]"

== system simTopLevel/Foot Trajectory Generation ==
  CPG In I : Inport
  CPG In II : Inport  Port=2
  CPG In III : Inport  Port=3
  CPG In IV : Inport  Port=4
  Leg I Trajectory : Outport
  Leg II Trajectory : Outport  Port=2
  Leg III Trajectory : Outport  Port=3
  Leg IV Trajectory : Outport  Port=4
  wires:
  CPG In I/1 -> Leg I Trajectory/1
  CPG In II/1 -> Leg II Trajectory/1
  CPG In III/1 -> Leg III Trajectory/1
  CPG In IV/1 -> Leg IV Trajectory/1

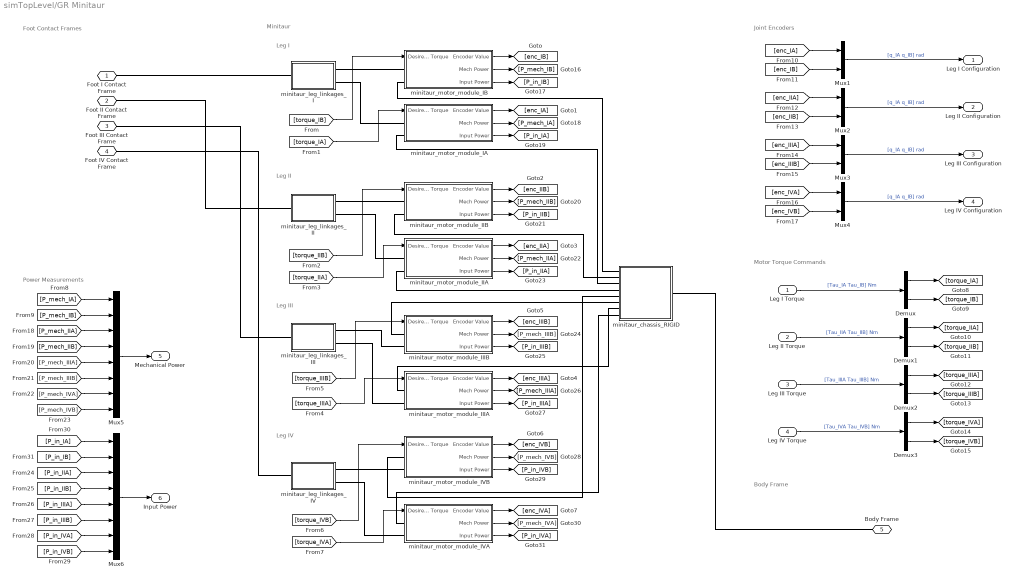
== system simTopLevel/GR Minitaur ==
  note: Minitaur
  note: Foot Contact Frames
  note: Joint Encoders
  note: Motor Torque Commands
  note: Body Frame
  note: Power Measurements
  note: Leg I
  note: Leg II
  note: Leg IV
  note: Leg III
  Leg I Torque : Inport
  Leg II Torque : Inport  Port=2
  Leg III Torque : Inport  Port=3
  Leg IV Torque : Inport  Port=4
  Demux{,1..3} (4 alike) : Demux  Outputs=2
  Mux{1..4} (4 alike) : Mux  Inputs=2
  Mux5 : Mux  Inputs=8
  Mux6 : Mux  Inputs=8
  minitaur_chassis_RIGID : Subsystem
  minitaur_leg_linkages_I : Subsystem
  minitaur_leg_linkages_II : Subsystem
  minitaur_leg_linkages_III : Subsystem
  minitaur_leg_linkages_IV : Subsystem
  minitaur_motor_module_IA : Subsystem
  minitaur_motor_module_IB : Subsystem
  minitaur_motor_module_IIA : Subsystem
  minitaur_motor_module_IIB : Subsystem
  minitaur_motor_module_IIIA : Subsystem
  minitaur_motor_module_IIIB : Subsystem
  minitaur_motor_module_IVA : Subsystem
  minitaur_motor_module_IVB : Subsystem
  Foot I Contact Frame : PMIOPort  Port=1  Side=Right
  Foot II Contact Frame : PMIOPort  Port=2  Side=Right
  Foot III Contact Frame : PMIOPort  Port=3  Side=Right
  Foot IV Contact Frame : PMIOPort  Port=4  Side=Right
  Body Frame : PMIOPort  Port=5  Side=Right
  Leg I Configuration : Outport
  Leg II Configuration : Outport  Port=2
  Leg III Configuration : Outport  Port=3
  Leg IV Configuration : Outport  Port=4
  Mechanical Power : Outport  Port=5
  Input Power : Outport  Port=6
  wires:
  Mux1/1 -> Leg I Configuration/1  "[q_IA q_IB] rad"
  Mux2/1 -> Leg II Configuration/1  "[q_IA q_IB] rad"
  Mux3/1 -> Leg III Configuration/1  "[q_IA q_IB] rad"
  Mux4/1 -> Leg IV Configuration/1  "[q_IA q_IB] rad"
  [enc_IB] -> Mux1/2
  [enc_IA] -> Mux1/1
  [enc_IIB] -> Mux2/2
  [enc_IIA] -> Mux2/1
  [enc_IIIB] -> Mux3/2
  [enc_IIIA] -> Mux3/1
  [enc_IVB] -> Mux4/2
  [enc_IVA] -> Mux4/1
  Leg IV Torque/1 -> Demux3/1  "[Tau_IVA Tau_IVB] Nm"
  Leg III Torque/1 -> Demux2/1  "[Tau_IIIA Tau_IIIB] Nm"
  Leg II Torque/1 -> Demux1/1  "[Tau_IIA Tau_IIB] Nm"
  Leg I Torque/1 -> Demux/1  "[Tau_IA Tau_IB] Nm"
  Demux/1 -> [torque_IA]
  Demux/2 -> [torque_IB]
  Demux1/1 -> [torque_IIA]
  Demux1/2 -> [torque_IIB]
  Demux2/1 -> [torque_IIIA]
  Demux2/2 -> [torque_IIIB]
  Demux3/1 -> [torque_IVA]
  Demux3/2 -> [torque_IVB]
  [P_mech_IB] -> Mux5/2
  [P_mech_IA] -> Mux5/1
  [P_mech_IIA] -> Mux5/3
  [P_mech_IIB] -> Mux5/4
  [P_mech_IIIA] -> Mux5/5
  [P_mech_IIIB] -> Mux5/6
  [P_mech_IVA] -> Mux5/7
  [P_mech_IVB] -> Mux5/8
  Mux5/1 -> Mechanical Power/1
  [P_in_IB] -> Mux6/2
  [P_in_IA] -> Mux6/1
  [P_in_IIA] -> Mux6/3
  [P_in_IIB] -> Mux6/4
  [P_in_IIIA] -> Mux6/5
  [P_in_IIIB] -> Mux6/6
  [P_in_IVA] -> Mux6/7
  [P_in_IVB] -> Mux6/8
  Mux6/1 -> Input Power/1
  minitaur_motor_module_IB/1(Encoder Value) -> [enc_IB]
  minitaur_motor_module_IA/1(Encoder Value) -> [enc_IA]
  [torque_IB] -> minitaur_motor_module_IB/1(Desired Torque)
  [torque_IA] -> minitaur_motor_module_IA/1(Desired Torque)
  minitaur_motor_module_IIB/1(Encoder Value) -> [enc_IIB]
  minitaur_motor_module_IIA/1(Encoder Value) -> [enc_IIA]
  [torque_IIB] -> minitaur_motor_module_IIB/1(Desired Torque)
  [torque_IIA] -> minitaur_motor_module_IIA/1(Desired Torque)
  [torque_IIIA] -> minitaur_motor_module_IIIA/1(Desired Torque)
  [torque_IIIB] -> minitaur_motor_module_IIIB/1(Desired Torque)
  minitaur_motor_module_IIIA/1(Encoder Value) -> [enc_IIIA]
  minitaur_motor_module_IIIB/1(Encoder Value) -> [enc_IIIB]
  [torque_IVA] -> minitaur_motor_module_IVA/1(Desired Torque)
  [torque_IVB] -> minitaur_motor_module_IVB/1(Desired Torque)
  minitaur_motor_module_IVB/1(Encoder Value) -> [enc_IVB]
  minitaur_motor_module_IB/3(Input Power) -> [P_in_IB]
  minitaur_motor_module_IB/2(Mech Power) -> [P_mech_IB]
  minitaur_motor_module_IA/2(Mech Power) -> [P_mech_IA]
  minitaur_motor_module_IA/3(Input Power) -> [P_in_IA]
  minitaur_motor_module_IIB/2(Mech Power) -> [P_mech_IIB]
  minitaur_motor_module_IIB/3(Input Power) -> [P_in_IIB]
  minitaur_motor_module_IIA/2(Mech Power) -> [P_mech_IIA]
  minitaur_motor_module_IIA/3(Input Power) -> [P_in_IIA]
  minitaur_motor_module_IIIB/2(Mech Power) -> [P_mech_IIIB]
  minitaur_motor_module_IIIB/3(Input Power) -> [P_in_IIIB]
  minitaur_motor_module_IIIA/2(Mech Power) -> [P_mech_IIIA]
  minitaur_motor_module_IIIA/3(Input Power) -> [P_in_IIIA]
  minitaur_motor_module_IVB/2(Mech Power) -> [P_mech_IVB]
  minitaur_motor_module_IVB/3(Input Power) -> [P_in_IVB]
  minitaur_motor_module_IVA/1(Encoder Value) -> [enc_IVA]
  minitaur_motor_module_IVA/2(Mech Power) -> [P_mech_IVA]
  minitaur_motor_module_IVA/3(Input Power) -> [P_in_IVA]
  connections:
  Foot II Contact Frame/RConn1 -- minitaur_leg_linkages_II/RConn1
  minitaur_leg_linkages_III/RConn1 -- Foot III Contact Frame/RConn1
  minitaur_chassis_RIGID/LConn8 -- minitaur_motor_module_IVA/LConn1
  minitaur_leg_linkages_I/LConn2 -- minitaur_motor_module_IA/LConn1
  minitaur_leg_linkages_I/LConn1 -- minitaur_motor_module_IB/LConn1
  minitaur_leg_linkages_IV/LConn2 -- minitaur_motor_module_IVA/LConn2
  minitaur_leg_linkages_III/LConn1 -- minitaur_motor_module_IIIB/LConn2
  minitaur_chassis_RIGID/LConn6 -- minitaur_motor_module_IIIB/LConn1
  minitaur_leg_linkages_II/LConn2 -- minitaur_motor_module_IIA/LConn1
  minitaur_leg_linkages_II/LConn1 -- minitaur_motor_module_IIB/LConn1
  minitaur_chassis_RIGID/LConn5 -- minitaur_motor_module_IVB/LConn1
  minitaur_chassis_RIGID/LConn4 -- minitaur_motor_module_IIA/LConn2
  minitaur_chassis_RIGID/LConn3 -- minitaur_motor_module_IA/LConn2
  minitaur_chassis_RIGID/LConn7 -- minitaur_motor_module_IIIA/LConn1
  minitaur_chassis_RIGID/LConn2 -- minitaur_motor_module_IIB/LConn2
  minitaur_chassis_RIGID/LConn1 -- minitaur_motor_module_IB/LConn2
  minitaur_leg_linkages_III/LConn2 -- minitaur_motor_module_IIIA/LConn2
  minitaur_leg_linkages_IV/LConn1 -- minitaur_motor_module_IVB/LConn2
  minitaur_chassis_RIGID/RConn1 -- Body Frame/RConn1
  minitaur_leg_linkages_I/RConn1 -- Foot I Contact Frame/RConn1
  minitaur_leg_linkages_IV/RConn1 -- Foot IV Contact Frame/RConn1

== system simTopLevel/Gait Timing // Leg Coordination Central Pattern Generator ==
  Constant{,1..3} (4 alike) : Constant  Value=[0 0]
  CPG Out I : Outport
  CPG Out II : Outport  Port=2
  CPG Out III : Outport  Port=3
  CPG Out IV : Outport  Port=4
  wires:
  Constant/1 -> CPG Out I/1
  Constant1/1 -> CPG Out II/1
  Constant2/1 -> CPG Out III/1
  Constant3/1 -> CPG Out IV/1

== system simTopLevel/Stop Conditions ==
  Body Position : Inport
  Fall Through Floor? : Fcn  Expr=u(3)<envParams.Ground.FrameDepth
  Fly Away? : Fcn  Expr=u(3)>envParams.Ground.FrameDepth+1.5
  Stop Simulation : Stop
  Stop Simulation1 : Stop
  wires:
  Fall Through Floor?/1 -> Stop Simulation/1
  Fly Away?/1 -> Stop Simulation1/1
  Body Position/1 -> Fly Away?/1, Fall Through Floor?/1

== system simTopLevel/Controller/Subsystem1 ==
  Path Trajectory : Inport
  Current leg state : Inport  Port=2
  Constant : Constant  Value=minitaurParams.Kinematics.L1
  Constant1 : Constant  Value=minitaurParams.Kinematics.L2
  Minitaur Leg Actuator Coordinates to Configuration Coordinates1 : MATLAB Function  TreatAsAtomicUnit=on
  Motor Angle PID : simulink/Continuous/PID Controller  Controller=PID  TimeDomain=Continuous-time  SampleTime=-1  IntegratorMethod=Forward Euler  FilterMethod=Forward Euler  Form=Parallel  UseFilter=on  ControllerParametersSource=internal  P=controlParams.jointPID.P  I=controlParams.jointPID.I  D=controlParams.jointPID.D  N=controlParams.jointPID.N  InitialConditionSource=internal  InitialConditionForIntegrator=0  InitialConditionForFilter=0  ExternalReset=none  LimitOutput=on  UpperSaturationLimit=inf  LowerSaturationLimit=-inf  LinearizeAsGain=on  AntiWindupMode=clamping  Kb=1  TrackingMode=off  Kt=1  PParamMin=[]  PParamMax=[]  IParamMin=[]  IParamMax=[]  DParamMin=[]  DParamMax=[]  NParamMin=[]  NParamMax=[]  KbParamMin=[]  KbParamMax=[]  KtParamMin=[]  KtParamMax=[]  POutMin=[]  POutMax=[]  IOutMin=[]  IOutMax=[]  DOutMin=[]  DOutMax=[]  NOutMin=[]  NOutMax=[]  KbOutMin=[]  KbOutMax=[]  KtOutMin=[]  KtOutMax=[]  IntegratorOutMin=[]  IntegratorOutMax=[]  FilterOutMin=[]  FilterOutMax=[]  SumOutMin=[]  SumOutMax=[]  SumI1OutMin=[]  SumI1OutMax=[]  SumI2OutMin=[]  SumI2OutMax=[]  SumI3OutMin=[]  SumI3OutMax=[]  SumDOutMin=[]  SumDOutMax=[]  SaturationOutMin=[]  SaturationOutMax=[]  IntegratorContinuousStateAttributes=''  IntegratorStateMustResolveToSignalObject=off  IntegratorRTWStateStorageClass=Auto  FilterContinuousStateAttributes=''  FilterStateMustResolveToSignalObject=off  FilterRTWStateStorageClass=Auto  DifferentiatorICPrevScaledInput=0  DifferentiatorOutMin=[]  DifferentiatorOutMax=[]
  Scope1 : Scope  NumInputPorts=2
  Scope2 : Scope
  Sum : Sum  Inputs=+-|
  Leg Torque : Outport
  wires:
  Sum/1 -> Motor Angle PID/1, Scope2/1  "[thetaA_err thetaB_err] rad"
  Current leg state/1 -> Sum/2, Scope1/2  "[thetaA,thetaB] rad"
  Motor Angle PID/1 -> Leg Torque/1
  Constant/1 -> Minitaur Leg Actuator Coordinates to Configuration Coordinates1/2(l1)
  Constant1/1 -> Minitaur Leg Actuator Coordinates to Configuration Coordinates1/3(l2)
  Path Trajectory/1 -> Minitaur Leg Actuator Coordinates to Configuration Coordinates1/1(a)
  Minitaur Leg Actuator Coordinates to Configuration Coordinates1/1(p) -> Scope1/1, Sum/1  "commanded [thetaA,thetaB] rad"

== system simTopLevel/Controller/Subsystem2 ==
  Path Trajectory : Inport
  Current leg state : Inport  Port=2
  Constant : Constant  Value=minitaurParams.Kinematics.L1
  Constant1 : Constant  Value=minitaurParams.Kinematics.L2
  Minitaur Leg Actuator Coordinates to Configuration Coordinates1 : MATLAB Function  TreatAsAtomicUnit=on
  Motor Angle PID : simulink/Continuous/PID Controller  Controller=PID  TimeDomain=Continuous-time  SampleTime=-1  IntegratorMethod=Forward Euler  FilterMethod=Forward Euler  Form=Parallel  UseFilter=on  ControllerParametersSource=internal  P=controlParams.jointPID.P  I=controlParams.jointPID.I  D=controlParams.jointPID.D  N=controlParams.jointPID.N  InitialConditionSource=internal  InitialConditionForIntegrator=0  InitialConditionForFilter=0  ExternalReset=none  LimitOutput=on  UpperSaturationLimit=inf  LowerSaturationLimit=-inf  LinearizeAsGain=on  AntiWindupMode=clamping  Kb=1  TrackingMode=off  Kt=1  PParamMin=[]  PParamMax=[]  IParamMin=[]  IParamMax=[]  DParamMin=[]  DParamMax=[]  NParamMin=[]  NParamMax=[]  KbParamMin=[]  KbParamMax=[]  KtParamMin=[]  KtParamMax=[]  POutMin=[]  POutMax=[]  IOutMin=[]  IOutMax=[]  DOutMin=[]  DOutMax=[]  NOutMin=[]  NOutMax=[]  KbOutMin=[]  KbOutMax=[]  KtOutMin=[]  KtOutMax=[]  IntegratorOutMin=[]  IntegratorOutMax=[]  FilterOutMin=[]  FilterOutMax=[]  SumOutMin=[]  SumOutMax=[]  SumI1OutMin=[]  SumI1OutMax=[]  SumI2OutMin=[]  SumI2OutMax=[]  SumI3OutMin=[]  SumI3OutMax=[]  SumDOutMin=[]  SumDOutMax=[]  SaturationOutMin=[]  SaturationOutMax=[]  IntegratorContinuousStateAttributes=''  IntegratorStateMustResolveToSignalObject=off  IntegratorRTWStateStorageClass=Auto  FilterContinuousStateAttributes=''  FilterStateMustResolveToSignalObject=off  FilterRTWStateStorageClass=Auto  DifferentiatorICPrevScaledInput=0  DifferentiatorOutMin=[]  DifferentiatorOutMax=[]
  Scope1 : Scope  NumInputPorts=2
  Scope2 : Scope
  Sum : Sum  Inputs=+-|
  Leg Torque : Outport
  wires:
  Sum/1 -> Motor Angle PID/1, Scope2/1  "[thetaA_err thetaB_err] rad"
  Current leg state/1 -> Sum/2, Scope1/2  "[thetaA,thetaB] rad"
  Motor Angle PID/1 -> Leg Torque/1
  Constant/1 -> Minitaur Leg Actuator Coordinates to Configuration Coordinates1/2(l1)
  Constant1/1 -> Minitaur Leg Actuator Coordinates to Configuration Coordinates1/3(l2)
  Path Trajectory/1 -> Minitaur Leg Actuator Coordinates to Configuration Coordinates1/1(a)
  Minitaur Leg Actuator Coordinates to Configuration Coordinates1/1(p) -> Scope1/1, Sum/1  "commanded [thetaA,thetaB] rad"

== system simTopLevel/Controller/Subsystem3 ==
  Path Trajectory : Inport
  Current leg state : Inport  Port=2
  Constant : Constant  Value=minitaurParams.Kinematics.L1
  Constant1 : Constant  Value=minitaurParams.Kinematics.L2
  Minitaur Leg Actuator Coordinates to Configuration Coordinates1 : MATLAB Function  TreatAsAtomicUnit=on
  Motor Angle PID : simulink/Continuous/PID Controller  Controller=PID  TimeDomain=Continuous-time  SampleTime=-1  IntegratorMethod=Forward Euler  FilterMethod=Forward Euler  Form=Parallel  UseFilter=on  ControllerParametersSource=internal  P=controlParams.jointPID.P  I=controlParams.jointPID.I  D=controlParams.jointPID.D  N=controlParams.jointPID.N  InitialConditionSource=internal  InitialConditionForIntegrator=0  InitialConditionForFilter=0  ExternalReset=none  LimitOutput=on  UpperSaturationLimit=inf  LowerSaturationLimit=-inf  LinearizeAsGain=on  AntiWindupMode=clamping  Kb=1  TrackingMode=off  Kt=1  PParamMin=[]  PParamMax=[]  IParamMin=[]  IParamMax=[]  DParamMin=[]  DParamMax=[]  NParamMin=[]  NParamMax=[]  KbParamMin=[]  KbParamMax=[]  KtParamMin=[]  KtParamMax=[]  POutMin=[]  POutMax=[]  IOutMin=[]  IOutMax=[]  DOutMin=[]  DOutMax=[]  NOutMin=[]  NOutMax=[]  KbOutMin=[]  KbOutMax=[]  KtOutMin=[]  KtOutMax=[]  IntegratorOutMin=[]  IntegratorOutMax=[]  FilterOutMin=[]  FilterOutMax=[]  SumOutMin=[]  SumOutMax=[]  SumI1OutMin=[]  SumI1OutMax=[]  SumI2OutMin=[]  SumI2OutMax=[]  SumI3OutMin=[]  SumI3OutMax=[]  SumDOutMin=[]  SumDOutMax=[]  SaturationOutMin=[]  SaturationOutMax=[]  IntegratorContinuousStateAttributes=''  IntegratorStateMustResolveToSignalObject=off  IntegratorRTWStateStorageClass=Auto  FilterContinuousStateAttributes=''  FilterStateMustResolveToSignalObject=off  FilterRTWStateStorageClass=Auto  DifferentiatorICPrevScaledInput=0  DifferentiatorOutMin=[]  DifferentiatorOutMax=[]
  Scope1 : Scope  NumInputPorts=2
  Scope2 : Scope
  Sum : Sum  Inputs=+-|
  Leg Torque : Outport
  wires:
  Sum/1 -> Motor Angle PID/1, Scope2/1  "[thetaA_err thetaB_err] rad"
  Current leg state/1 -> Sum/2, Scope1/2  "[thetaA,thetaB] rad"
  Motor Angle PID/1 -> Leg Torque/1
  Constant/1 -> Minitaur Leg Actuator Coordinates to Configuration Coordinates1/2(l1)
  Constant1/1 -> Minitaur Leg Actuator Coordinates to Configuration Coordinates1/3(l2)
  Path Trajectory/1 -> Minitaur Leg Actuator Coordinates to Configuration Coordinates1/1(a)
  Minitaur Leg Actuator Coordinates to Configuration Coordinates1/1(p) -> Scope1/1, Sum/1  "commanded [thetaA,thetaB] rad"

== system simTopLevel/Controller/Subsystem4 ==
  Path Trajectory : Inport
  Current leg state : Inport  Port=2
  Constant : Constant  Value=minitaurParams.Kinematics.L1
  Constant1 : Constant  Value=minitaurParams.Kinematics.L2
  Minitaur Leg Actuator Coordinates to Configuration Coordinates1 : MATLAB Function  TreatAsAtomicUnit=on
  Motor Angle PID : simulink/Continuous/PID Controller  Controller=PID  TimeDomain=Continuous-time  SampleTime=-1  IntegratorMethod=Forward Euler  FilterMethod=Forward Euler  Form=Parallel  UseFilter=on  ControllerParametersSource=internal  P=controlParams.jointPID.P  I=controlParams.jointPID.I  D=controlParams.jointPID.D  N=controlParams.jointPID.N  InitialConditionSource=internal  InitialConditionForIntegrator=0  InitialConditionForFilter=0  ExternalReset=none  LimitOutput=on  UpperSaturationLimit=inf  LowerSaturationLimit=-inf  LinearizeAsGain=on  AntiWindupMode=clamping  Kb=1  TrackingMode=off  Kt=1  PParamMin=[]  PParamMax=[]  IParamMin=[]  IParamMax=[]  DParamMin=[]  DParamMax=[]  NParamMin=[]  NParamMax=[]  KbParamMin=[]  KbParamMax=[]  KtParamMin=[]  KtParamMax=[]  POutMin=[]  POutMax=[]  IOutMin=[]  IOutMax=[]  DOutMin=[]  DOutMax=[]  NOutMin=[]  NOutMax=[]  KbOutMin=[]  KbOutMax=[]  KtOutMin=[]  KtOutMax=[]  IntegratorOutMin=[]  IntegratorOutMax=[]  FilterOutMin=[]  FilterOutMax=[]  SumOutMin=[]  SumOutMax=[]  SumI1OutMin=[]  SumI1OutMax=[]  SumI2OutMin=[]  SumI2OutMax=[]  SumI3OutMin=[]  SumI3OutMax=[]  SumDOutMin=[]  SumDOutMax=[]  SaturationOutMin=[]  SaturationOutMax=[]  IntegratorContinuousStateAttributes=''  IntegratorStateMustResolveToSignalObject=off  IntegratorRTWStateStorageClass=Auto  FilterContinuousStateAttributes=''  FilterStateMustResolveToSignalObject=off  FilterRTWStateStorageClass=Auto  DifferentiatorICPrevScaledInput=0  DifferentiatorOutMin=[]  DifferentiatorOutMax=[]
  Scope1 : Scope  NumInputPorts=2
  Scope2 : Scope
  Sum : Sum  Inputs=+-|
  Leg Torque : Outport
  wires:
  Sum/1 -> Motor Angle PID/1, Scope2/1  "[thetaA_err thetaB_err] rad"
  Current leg state/1 -> Sum/2, Scope1/2  "[thetaA,thetaB] rad"
  Motor Angle PID/1 -> Leg Torque/1
  Constant/1 -> Minitaur Leg Actuator Coordinates to Configuration Coordinates1/2(l1)
  Constant1/1 -> Minitaur Leg Actuator Coordinates to Configuration Coordinates1/3(l2)
  Path Trajectory/1 -> Minitaur Leg Actuator Coordinates to Configuration Coordinates1/1(a)
  Minitaur Leg Actuator Coordinates to Configuration Coordinates1/1(p) -> Scope1/1, Sum/1  "commanded [thetaA,thetaB] rad"
